simulink model "hvac_pid_heating_and_cooling"  (R2024a)
settings: Solver=FixedStepDiscrete  StartTime=0.0  StopTime=simStopTime  FixedStep=sampleTimeSeconds  RelTol=1e-3
undefined symbols (not defined in the file): a, b_cool, b_heat, c, sampleTimeSeconds, T0
libraries: slpidlib x1
settings Model: Creator=saimh  LastModifiedBy=saimh

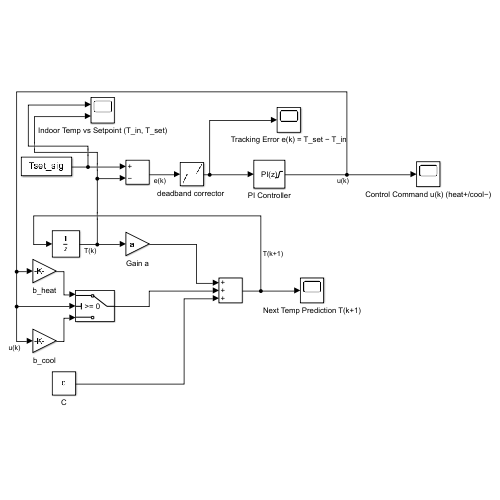
[thumbnail: Simulink's stored preview of the top-level diagram]
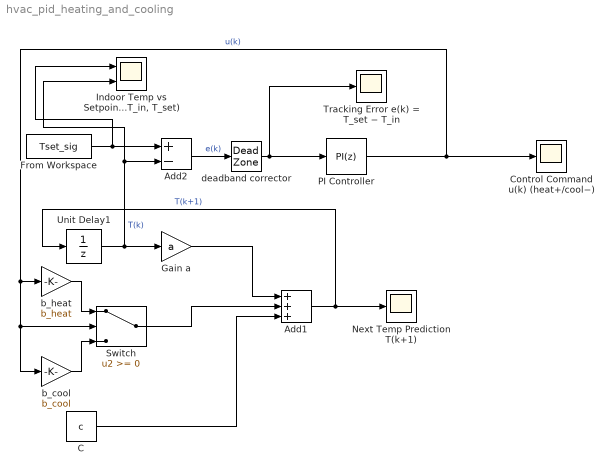
== system hvac_pid_heating_and_cooling ==
  Add1 : Sum  Inputs=+++
  Add2 : Sum  Inputs=+-
  C : Constant  Value=c
  Control Command u(k) (heat+/cool−) : Scope
  From Workspace : FromWorkspace  VariableName=Tset_sig  SampleTime=sampleTimeSeconds  Interpolate=off  OutputAfterFinalValue=Holding final value
  Gain a : Gain  Gain=a
  "Indoor Temp vs Setpoint (T_in, T_set)" : Scope  NumInputPorts=2
  Next Temp Prediction T(k+1) : Scope
  PI Controller : slpidlib/PID Controller  Controller=PI  Form=Parallel  TimeDomain=Discrete-time  UseExternalTs=off  SampleTime=sampleTimeSeconds  IntegratorMethod=Backward Euler  FilterMethod=Forward Euler  ControllerParametersSource=internal  P=0.9  I=1.75e-5  UseKiTs=off  D=0  UseExternalDerivativeSource=off  N=100  UseFilter=on  TunerSelectOption=Transfer Function Based (PID Tuner App)  ZeroCross=off  InitialConditionSource=internal  InitialConditionForIntegrator=0  InitialConditionForFilter=0  DifferentiatorICPrevScaledInput=0  ExternalReset=none  TrackingMode=off  Kt=1  LimitOutput=on  SatLimitsSource=internal  UpperSaturationLimit=1  LowerSaturationLimit=-1  LinearizeAsGain=off  AntiWindupMode=back-calculation  Kb=2  LimitIntegrator=on  UpperIntegratorSaturationLimit=1  LowerIntegratorSaturationLimit=-1  POutMin=[]  POutMax=[]  IOutMin=[]  IOutMax=[]  DOutMin=[]  DOutMax=[]  NOutMin=[]  NOutMax=[]  SumOutMin=[]  SumOutMax=[]  SaturationOutMin=[]  SaturationOutMax=[]  PParamMin=[]  PParamMax=[]  IParamMin=[]  IParamMax=[]  DParamMin=[]  DParamMax=[]  NParamMin=[]  NParamMax=[]  KbParamMin=[]  KbParamMax=[]  KtParamMin=[]  KtParamMax=[]  KbOutMin=[]  KbOutMax=[]  KtOutMin=[]  KtOutMax=[]  IntegratorOutMin=[]  IntegratorOutMax=[]  FilterOutMin=[]  FilterOutMax=[]  SumI1OutMin=[]  SumI1OutMax=[]  SumI2OutMin=[]  SumI2OutMax=[]  SumI3OutMin=[]  SumI3OutMax=[]  SumI4OutMin=[]  SumI4OutMax=[]  SumDOutMin=[]  SumDOutMax=[]  DifferentiatorOutMin=[]  DifferentiatorOutMax=[]  FilterDiffOutCoefMin=[]  FilterDiffOutCoefMax=[]  ReciprocalOutMin=[]  ReciprocalOutMax=[]  SumDenOutMin=[]  SumDenOutMax=[]  SumNumOutMin=[]  SumNumOutMax=[]  DivideOutMin=[]  DivideOutMax=[]  UdiffTsProdOutMin=[]  UdiffTsProdOutMax=[]  NTsProdOutMin=[]  NTsProdOutMax=[]  UintegralTsProdOutMin=[]  UintegralTsProdOutMax=[]  UngainTsProdOutMin=[]  UngainTsProdOutMax=[]  ClampingZeroOutDataTypeStr=Inherit: Inherit via back propagation  ClampingZeroOutMin=[]  ClampingZeroOutMax=[]  FilterDenConstantOutDataTypeStr=Inherit: Inherit via back propagation  FilterDenConstantOutMin=[]  FilterDenConstantOutMax=[]  PCopyOutDataTypeStr=Inherit: Inherit via back propagation  PCopyOutMin=[]  PCopyOutMax=[]  NCopyOutDataTypeStr=Inherit: Inherit via back propagation  NCopyOutMin=[]  NCopyOutMax=[]  IntegratorContinuousStateAttributes=''  IntegratorStateMustResolveToSignalObject=off  IntegratorRTWStateStorageClass=Auto  FilterContinuousStateAttributes=''  FilterStateMustResolveToSignalObject=off  FilterRTWStateStorageClass=Auto  ParallelPVariant=InternalParameters  IdealPVariant=Disabled  IVariant=InternalParameters  DVariant=Disabled  IntegratorVariant=Discrete  SatVariant=Enabled  AWVariant=BackCalculation  PCopyVariant=Disabled  TRVariant=Disabled  FdbkBlocksVariant=Feedback  IdealPFdbkVariant=Passthrough  SatFdbkVariant=Enabled  DerivativeFilterVariant=Disabled  NVariant=Disabled  NCopyVariant=Disabled_SignalSpec  FilterICVariant=Disabled  IntegratorICVariant=InternalICs  ExternalResetVariant=Disabled  TRSumVariant=Passthrough  SumFdbkVariant=Enabled  SumVariant=Sum_PI  TsampFilterVariant=InternalTs  TsampNgainVariant=Passthrough  TsampIntegralVariant=Disabled_SignalSpec  ExternalSaturationOutDataTypeStr=Inherit: Same as second input  DerivativeSourceVariant=Disabled
      settings: LibrarySourceBlock=simulink/Discrete/Discrete PID Controller
  Switch : Switch  SaturateOnIntegerOverflow=off  InputSameDT=off
  Tracking Error e(k) = T_set − T_in : Scope
  Unit Delay1 : UnitDelay  InitialCondition=T0  SampleTime=sampleTimeSeconds  HasFrameUpgradeWarning=on
  b_cool : Gain  Gain=b_cool
  b_heat : Gain  Gain=b_heat
  "deadband corrector " : DeadZone  LowerValue=-0.25  UpperValue=0.25
  wires:
  Unit Delay1/1 -> Gain a/1, "Indoor Temp vs Setpoint (T_in, T_set)"/2, Add2/2  "T(k)"
  Gain a/1 -> Add1/1
  Switch/1 -> Add1/2
  C/1 -> Add1/3
  Add1/1 -> Next Temp Prediction T(k+1)/1, Unit Delay1/1  "T(k+1)"
  From Workspace/1 -> "Indoor Temp vs Setpoint (T_in, T_set)"/1, Add2/1
  Add2/1 -> "deadband corrector "/1  "e(k)"
  PI Controller/1 -> Switch/2, b_cool/1, b_heat/1, Control Command u(k) (heat+/cool−)/1  "u(k)"
  b_heat/1 -> Switch/1
  b_cool/1 -> Switch/3
  "deadband corrector "/1 -> PI Controller/1, Tracking Error e(k) = T_set − T_in/1
